simulink model "ch7example26"  (Simulink 5.0)
settings: Solver=ode45  StartTime=0.0  StopTime=1000.0  MaxStep=1e-4  RelTol=1e-3
undefined symbols (not defined in the file): Fs
libraries: commutil2 x5, simulink x4, dspsnks4 x3, commdigbbndpm2 x2, commrandsrc2 x2, commseqgen2 x2, commchan2 x1, commsink2 x1, dspsigops x1
settings Model: LastModifiedBy=shaoyubin

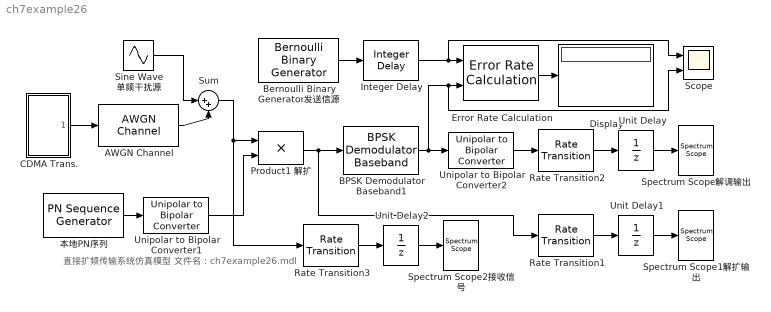
== system ch7example26 ==
  note: 直接扩频传输系统仿真模型
      | 文件名：ch7example26.mdl
  AWGN Channel : commchan2/AWGN Channel  seed=67  noiseMode=Variance from mask  EsNodB=10  SNRdB=10  Ps=1  Tsym=1  variance=10
  BPSK Demodulator Baseband1 : commdigbbndpm2/BPSK Demodulator Baseband  Ph=0  numSamp=20
  Bernoulli Binary Generator发送信源 : commrandsrc2/Bernoulli Binary Generator  P=0.5  seed=61  Ts=1/100  frameBased=off  sampPerFrame=1  orient=off
  CDMA Trans. : Subsystem
  Display : Display
  Error Rate Calculation : commsink2/Error Rate Calculation  N=0  st_delay=0  cp_mode=Entire frame  subframe=[]  PMode=Port  WsName=ErrorVec  RsMode2=off  stop=off  numErr=100  maxBits=1e6
  Integer Delay : dspsigops/Integer Delay  delay=2  ic=0  reset_popup=None
  Product1 解扩 : Product  SaturateOnIntegerOverflow=on
  Rate Transition1 : simulink/Signal Attributes/Rate Transition  DataIntegrity=on  DeterministicTransfer=on  TransitionType=Slow to fast  InitCond=0
  Rate Transition2 : simulink/Signal Attributes/Rate Transition  DataIntegrity=on  DeterministicTransfer=on  TransitionType=Slow to fast  InitCond=0
  Rate Transition3 : simulink/Signal Attributes/Rate Transition  DataIntegrity=on  DeterministicTransfer=on  TransitionType=Slow to fast  InitCond=0
  Scope : Scope  NumInputPorts=2
      settings: TimeRange=0.4  YMin=-2~-2  YMax=2~2
  Sine Wave 单频干扰源 : Sin  Frequency=2*pi*300  SampleTime=1/2000
  Spectrum Scope1解扩输出 : dspsnks4/Spectrum Scope  ScopeProperties=off  Domain=Frequency  HorizSpan=1  UseBuffer=on  BufferSize=1024  Overlap=512  inpFftLenInherit=on  FFTlength=1024  numAvg=500  DisplayProperties=off  AxisGrid=on  Memory=off  FrameNumber=on  AxisLegend=off  AxisZoom=off  OpenScopeAtSimStart=on  OpenScopeImmediately=off  FigPos=[232 258 560 420]  AxisProperties=on  XUnits=Hertz  XRange=[-Fs/2...Fs/2]  InheritXIncr=on  XIncr=1  XLabel=Samples  YUnits=dB  YLabel=Magnitude, dB  LineProperties=off  LineMarkers=|None  LineColors=|[1 0 0]
      settings: YMin=-40  YMax=25
  Spectrum Scope2接收信号 : dspsnks4/Spectrum Scope  ScopeProperties=off  Domain=Frequency  HorizSpan=1  UseBuffer=on  BufferSize=1024  Overlap=512  inpFftLenInherit=on  FFTlength=1024  numAvg=500  DisplayProperties=off  AxisGrid=on  Memory=off  FrameNumber=on  AxisLegend=off  AxisZoom=off  OpenScopeAtSimStart=on  OpenScopeImmediately=off  FigPos=[232 258 560 420]  AxisProperties=on  XUnits=Hertz  XRange=[-Fs/2...Fs/2]  InheritXIncr=on  XIncr=1  XLabel=Samples  YUnits=dB  YLabel=Magnitude, dB  LineProperties=off  LineMarkers=|None  LineColors=|[0 0 1]
      settings: YMin=-40  YMax=25
  Spectrum Scope解调输出 : dspsnks4/Spectrum Scope  ScopeProperties=off  Domain=Frequency  HorizSpan=1  UseBuffer=on  BufferSize=1024  Overlap=512  inpFftLenInherit=on  FFTlength=1024  numAvg=500  DisplayProperties=off  AxisGrid=on  Memory=off  FrameNumber=on  AxisLegend=off  AxisZoom=off  OpenScopeAtSimStart=on  OpenScopeImmediately=off  FigPos=[232 258 560 420]  AxisProperties=on  XUnits=Hertz  XRange=[-Fs/2...Fs/2]  InheritXIncr=on  XIncr=1  XLabel=Samples  YUnits=dB  YLabel=Magnitude, dB  LineProperties=off  LineMarkers=|None  LineColors=|[1 0 0]
      settings: YMin=-40  YMax=25
  Sum : Sum  Inputs=|++  SaturateOnIntegerOverflow=on
  Unipolar to Bipolar Converter1 : commutil2/Unipolar to Bipolar Converter  M=2  polarity=Positive
  Unipolar to Bipolar Converter2 : commutil2/Unipolar to Bipolar Converter  M=2  polarity=Positive
  Unit Delay : UnitDelay  SampleTime=1/8000
  Unit Delay1 : UnitDelay  SampleTime=1/8000
  Unit Delay2 : UnitDelay  SampleTime=1/8000
  本地PN序列 : commseqgen2/PN Sequence Generator  poly=[1 0 0 0 0 1 1]  ini_sta=[0 0 0 0 0 1]  shift=0  Ts=1/2000  frameBased=off  sampPerFrame=1  reset=off
  wires:
  Unit Delay/1 -> Spectrum Scope解调输出/1
  Rate Transition2/1 -> Unit Delay/1
  CDMA Trans./1(CDMA) -> AWGN Channel/1
  Unit Delay1/1 -> Spectrum Scope1解扩输出/1
  Rate Transition1/1 -> Unit Delay1/1
  本地PN序列/1 -> Unipolar to Bipolar Converter1/1
  Unipolar to Bipolar Converter1/1 -> Product1 解扩/2
  Product1 解扩/1 -> BPSK Demodulator Baseband1/1, Rate Transition1/1
  BPSK Demodulator Baseband1/1 -> Unipolar to Bipolar Converter2/1, Error Rate Calculation/2, Scope/2
  Unipolar to Bipolar Converter2/1 -> Rate Transition2/1
  Bernoulli Binary Generator发送信源/1 -> Integer Delay/1
  Integer Delay/1 -> Error Rate Calculation/1, Scope/1
  Error Rate Calculation/1 -> Display/1
  Unit Delay2/1 -> Spectrum Scope2接收信号/1
  Rate Transition3/1 -> Unit Delay2/1
  Sum/1 -> Product1 解扩/1, Rate Transition3/1
  AWGN Channel/1 -> Sum/2
  Sine Wave 单频干扰源/1 -> Sum/1

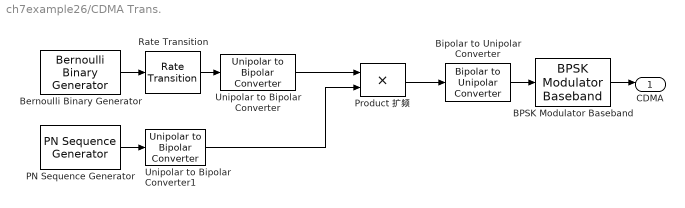
== system ch7example26/CDMA Trans. ==
  BPSK Modulator Baseband : commdigbbndpm2/BPSK Modulator Baseband  Ph=0  numSamp=1
  Bernoulli Binary Generator : commrandsrc2/Bernoulli Binary Generator  P=0.5  seed=61  Ts=1/100  frameBased=off  sampPerFrame=1  orient=off
  Bipolar to Unipolar Converter : commutil2/Bipolar to Unipolar Converter  M=2  polarity=Positive
  PN Sequence Generator : commseqgen2/PN Sequence Generator  poly=[1 0 0 0 0 1 1]  ini_sta=[0 0 0 0 0 1]  shift=0  Ts=1/2000  frameBased=off  sampPerFrame=1  reset=off
  Product 扩频 : Product  SaturateOnIntegerOverflow=on
  Rate Transition : simulink/Signal Attributes/Rate Transition  DataIntegrity=on  DeterministicTransfer=on  TransitionType=Slow to fast  InitCond=0
  Unipolar to Bipolar Converter : commutil2/Unipolar to Bipolar Converter  M=2  polarity=Positive
  Unipolar to Bipolar Converter1 : commutil2/Unipolar to Bipolar Converter  M=2  polarity=Positive
  CDMA : Outport
  wires:
  Bernoulli Binary Generator/1 -> Rate Transition/1
  PN Sequence Generator/1 -> Unipolar to Bipolar Converter1/1
  Product 扩频/1 -> Bipolar to Unipolar Converter/1
  Unipolar to Bipolar Converter/1 -> Product 扩频/1
  Bipolar to Unipolar Converter/1 -> BPSK Modulator Baseband/1
  Unipolar to Bipolar Converter1/1 -> Product 扩频/2
  Rate Transition/1 -> Unipolar to Bipolar Converter/1
  BPSK Modulator Baseband/1 -> CDMA/1
